simulink model "ReadLidar"  (R2015a)
settings: Solver=FixedStepDiscrete  StartTime=0.0  StopTime=inf  FixedStep=.0001  RelTol=1e-3
PreSaveFcn:
  | set_param(gcs, 'location', [15 50 815 560])
settings Model: SimulationMode=external  ExtModeTrigDuration=100  Creator=The MathWorks Inc.  LastModifiedBy=Will
settings DataIOCC: SignalLoggingSaveFormat=ModelDataLogs
settings OptimizationCC: ExpressionDepthLimit=2147483647  OptimizeModelRefInitCode=on  LifeSpan=Inf
settings DebuggingCC: UnderspecifiedInitializationDetection=Classic  MergeDetectMultiDrivingBlocksExec=none  FcnCallInpInsideContextMsg=EnableAllAsWarning  StateNameClashWarn=warning
settings HardwareCC: ProdLargestAtomicInteger=Long  ProdLargestAtomicFloat=Double  ProdEndianess=LittleEndian  ProdHWDeviceType=ARM Compatible->ARM Cortex
settings RTWCC: SystemTargetFile=realtime.tlc  GenerateMakefile=off  TemplateMakefile=realtime.tmf  Description=Run on Target Hardware  RTWVerbose=off  CustomInclude=/home/pi/wiringPi/wiringPi/
settings CodeAppCC: CustomSymbolStrType=$N$R$M  InternalIdentifier=Classic
settings ERTTargetCC: CombineOutputUpdateFcns=off  ExtMode=on  ExtModeMexArgs='192.168.2.5' 0 17725  ERTSrcFileBannerTemplate=realtime_code_template.cgt  ERTHdrFileBannerTemplate=realtime_code_template.cgt  ERTDataSrcFileTemplate=realtime_code_template.cgt  ERTDataHdrFileTemplate=realtime_code_template.cgt  ERTCustomFileTemplate=realtime_file_process.tlc

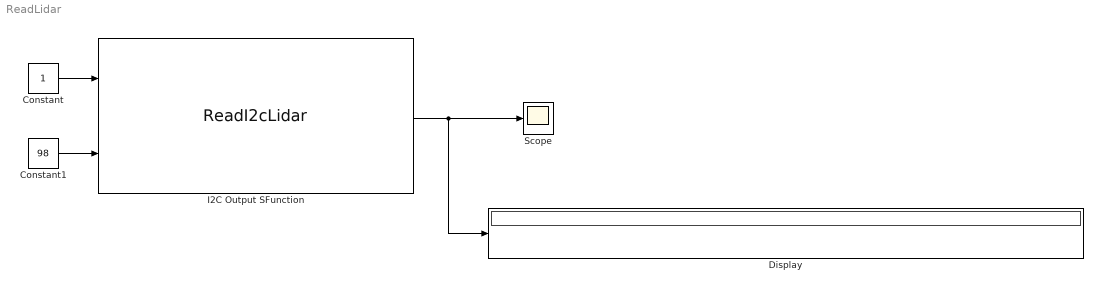
== system ReadLidar ==
  Constant : Constant  OutDataTypeStr=uint8
  Constant1 : Constant  Value=98  OutDataTypeStr=uint8
  Display : Display
  I2C Output SFunction : S-Function  InitFcn=try, set_param(gcb,'FunctionName','ReadI2cLidar'), end  FunctionName=ReadI2cLidar  SFunctionModules=ReadI2cLidar_wrapper  mask(S-Function Builder){}
      mask init:
      | val = [[.9  0.75 0.75 1 1 .9 .9 1]',[1 1 0.75 0.75 .9 .9 1 .9]'];try , sys = get_param(gcb,'SfunBuilderFcnName');if isempty(sys), sys = get_param(gcb,'FunctionName'); end,catch, sys = get_param(gcb,'FunctionName'); end
      settings: CopyFcn=set_param(gcbh,'LinkStatus','none')  PreSaveFcn=try, set_param(gcb,'FunctionName','ReadI2cLidar'), end  OpenFcn=sfunctionwizard(gcbh)
      mask Display: plot(val(:,1),val(:,2)),disp(sys), port_label('input',1,'Bus_Number'), port_label('input',2,'Device_Address'), port_label('output',1,'Register_Value')
  Scope : Scope
      settings: YMin=0  YMax=1300
  wires:
  I2C Output SFunction/1 -> Display/1, Scope/1
  Constant/1 -> I2C Output SFunction/1
  Constant1/1 -> I2C Output SFunction/2
